simulink model "bprz"  (R2021a)
settings: Solver=VariableStepAuto  StartTime=0.0  StopTime=10.0  RelTol=1e-3
libraries: commrandsrc3 x1, commutil2 x1
settings Model: Creator=ASUS  LastModifiedBy=ASUS

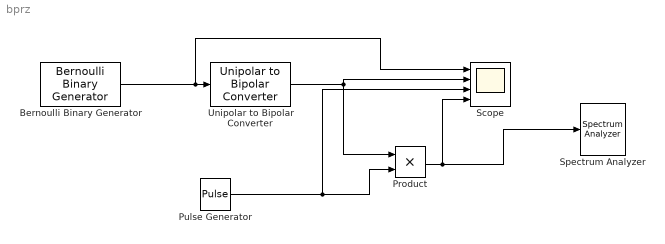
== system bprz ==
  Bernoulli Binary Generator : commrandsrc3/Bernoulli Binary Generator  ProbabilityOfZero=0.5  SeedSource=Parameter  Seed=61  SampleTime=0.0001  SamplesPerFrame=1  OutputDataType=double  SimulateUsing=Interpreted execution
  Product : Product
  Pulse Generator : DiscretePulseGenerator  Period=10  PulseWidth=5  SampleTime=0.00001
  Scope : Scope  NumInputPorts=4
  Spectrum Analyzer : SpectrumAnalyzer
  Unipolar to Bipolar Converter : commutil2/Unipolar to Bipolar Converter  M=2  polarity=Positive  dataType=Inherit via internal rule
  wires:
  Bernoulli Binary Generator/1 -> Scope/1, Unipolar to Bipolar Converter/1
  Unipolar to Bipolar Converter/1 -> Scope/2, Product/1
  Pulse Generator/1 -> Scope/3, Product/2
  Product/1 -> Scope/4, Spectrum Analyzer/1
